simulink model "Room_Eq"  (R2024b)
settings: Solver=VariableStepAuto  StartTime=0.0  StopTime=20  RelTol=1e-3
libraries: dspvision x3, dspsnks4 x2, dspadpt3 x1
settings Model: Creator=tamiz  LastModifiedBy=tamiz

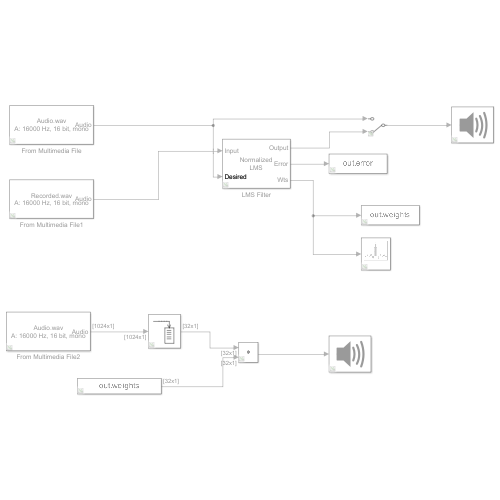
[thumbnail: Simulink's stored preview of the top-level diagram]
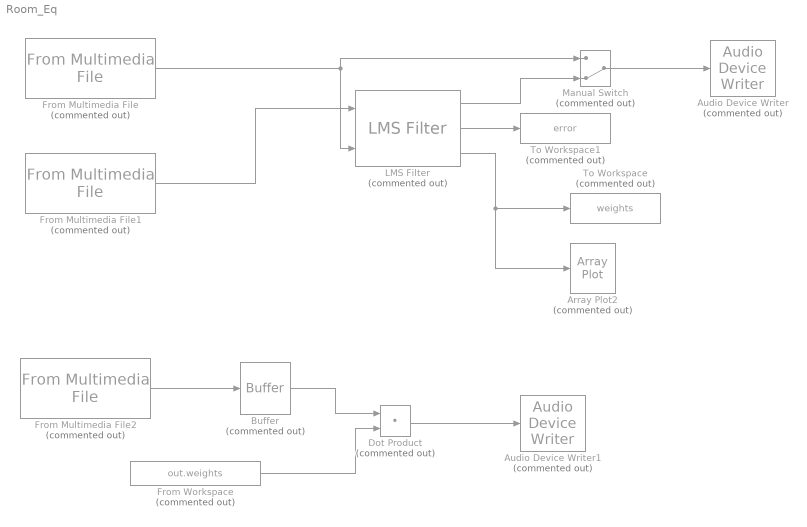
== system Room_Eq ==
  Array Plot2 : ArrayPlot  Commented=on  WindowPosition=[311.000000,280.000000,800.000000,500.000000,]  ScopeFrameLocation=window  YLimits=[-0.494 0.5139]
      settings: OpenAtSimulationStart=off
  Audio Device Writer : dspsnks4/Audio Device Writer  Commented=on  Driver=DirectSound  Device=Default  InheritSampleRate=on  SampleRate=44100  BitDepth=16-bit integer  BufferSize=4096  NumBuffers=10  DefaultOutputChannelMapping=on  OutputChannelMapping=1:2  OutputNumUnderrunSamples=off  DriverIdx=1  DeviceWarnFlag=''
  Audio Device Writer1 : dspsnks4/Audio Device Writer  Commented=on  Driver=DirectSound  Device=Default  InheritSampleRate=on  SampleRate=44100  BitDepth=16-bit integer  BufferSize=4096  NumBuffers=10  DefaultOutputChannelMapping=on  OutputChannelMapping=1:2  OutputNumUnderrunSamples=off  DriverIdx=1  DeviceWarnFlag=''
  Buffer : Buffer  Commented=on  N=32  V=31  OutputFrames=off
  Dot Product : DotProduct  Commented=on  OutDataTypeStr=Inherit: Inherit via internal rule
  From Workspace : FromWorkspace  Commented=on  VariableName=out.weights
  From Multimedia File : dspvision/From Multimedia File  Commented=on  inputFilename=C:\Users\tamiz\Documents\IITGN\6th_sem\ASP\Project_1\Audio.wav  readRange=[1 Inf]  loop=on  numPlays=inf  outputStreams=Audio only  videoDataType=single  audioDataType=double  inheritSampleTime=on  userDefinedSampleTime=1/30  noAudioOutput=off  isIntensityVideo=off  fourcc=RGB  colorVideoFormat=One multidimensional signal  outputEOF=off  dataOrg=Column-major  audioFrameSize=1024  computeAudioFrameSize=off  outSamplingMode=Sample based
      settings: LibrarySourceBlock=dspsrcs4/From Multimedia File
  From Multimedia File1 : dspvision/From Multimedia File  Commented=on  inputFilename=C:\Users\tamiz\Documents\IITGN\6th_sem\ASP\Project_1\Recorded.wav  readRange=[1 Inf]  loop=on  numPlays=inf  outputStreams=Audio only  videoDataType=single  audioDataType=double  inheritSampleTime=on  userDefinedSampleTime=1/30  noAudioOutput=off  isIntensityVideo=off  fourcc=RGB  colorVideoFormat=One multidimensional signal  outputEOF=off  dataOrg=Column-major  audioFrameSize=1024  computeAudioFrameSize=off  outSamplingMode=Sample based
      settings: LibrarySourceBlock=dspsrcs4/From Multimedia File
  From Multimedia File2 : dspvision/From Multimedia File  Commented=on  inputFilename=C:\Users\tamiz\Documents\IITGN\6th_sem\ASP\Project_1\Audio.wav  readRange=[1 Inf]  loop=on  numPlays=inf  outputStreams=Audio only  videoDataType=single  audioDataType=double  inheritSampleTime=on  userDefinedSampleTime=1/30  noAudioOutput=off  isIntensityVideo=off  fourcc=RGB  colorVideoFormat=One multidimensional signal  outputEOF=off  dataOrg=Column-major  audioFrameSize=1024  computeAudioFrameSize=off  outSamplingMode=Sample based
      settings: LibrarySourceBlock=dspsrcs4/From Multimedia File
  LMS Filter : dspadpt3/LMS Filter  Commented=on  Algo=Normalized LMS  L=32  stepflag=Dialog  mu=0.01  leakage=1.0  ic=0  Adapt=off  resetflag=None  weights=on  addnparflag=off  roundingMode=Floor  overflowMode=off  secondCoeffMode=Binary point scaling  secondCoeffWordLength=2  secondCoeffFracLength=15  prodOutput2Mode=Binary point scaling  prodOutput2FracLength=20  prodOutput3Mode=Binary point scaling  prodOutput3FracLength=20  prodOutput4Mode=Binary point scaling  prodOutput4FracLength=20  quotientMode=Binary point scaling  quotientFracLength=20  accum2Mode=Binary point scaling  accum2FracLength=20
      settings: LibrarySourceBlock=dsphdlsupportfiltering/LMS Filter
  Manual Switch : ManualSwitch  Commented=on  CurrentSetting=0
  To Workspace : ToWorkspace  Commented=on  VariableName=weights  SaveFormat=Timeseries  SampleTime=-1
      settings: MaxDataPoints=32  Save2DSignal=2-D array (concatenate along first dimension)
  To Workspace1 : ToWorkspace  Commented=on  VariableName=error  SampleTime=-1
      settings: Save2DSignal=2-D array (concatenate along first dimension)
  wires:
  From Multimedia File/1 -> Manual Switch/1, LMS Filter/2
  From Multimedia File1/1 -> LMS Filter/1
  Manual Switch/1 -> Audio Device Writer/1
  LMS Filter/3 -> To Workspace/1, Array Plot2/1
  LMS Filter/1 -> Manual Switch/2
  LMS Filter/2 -> To Workspace1/1
  From Multimedia File2/1 -> Buffer/1
  Buffer/1 -> Dot Product/1
  From Workspace/1 -> Dot Product/2
  Dot Product/1 -> Audio Device Writer1/1
